simulink model "ss_feedback"  (R2022a)
settings: Solver=VariableStepAuto  StartTime=0.0  StopTime=100  RelTol=1e-3
values from neighbouring files (symbols this model uses):
  B = [0 2]'    [delayIndependent_Razumikhin_analysis.m]
  C = eye(2)    [delayIndependent_Razumikhin_synthesis.m]
  K = -[0.9 0]    [delayIndependent_Razumikhin_analysis.m]    (also in delayIndependent_Razumikhin_synthesis.m = Y*P)
undefined symbols (not defined in the file or in its folder): A
settings Model: Creator=aaron  LastModifiedBy=aaron

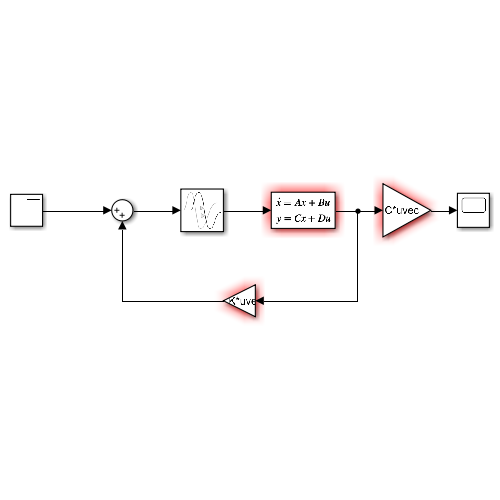
[thumbnail: Simulink's stored preview of the top-level diagram]
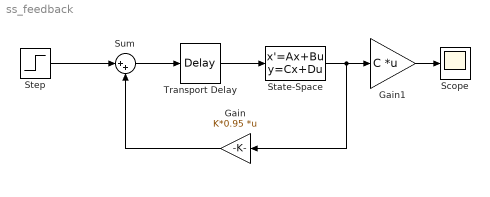
== system ss_feedback ==
  Gain : Gain  Gain=K*0.95  Multiplication=Matrix(K*u) (u vector)
  Gain1 : Gain  Gain=C  Multiplication=Matrix(K*u) (u vector)
  Scope : Scope
  State-Space : StateSpace  A=A  B=B  C=eye(2)  D=zeros(2,1)  InitialCondition=0
  Step : Step  Time=0  SampleTime=0
  Sum : Sum  Inputs=|++
  Transport Delay : TransportDelay  DelayTime=10
  wires:
  Transport Delay/1 -> State-Space/1
  State-Space/1 -> Gain/1, Gain1/1
  Step/1 -> Sum/1
  Sum/1 -> Transport Delay/1
  Gain/1 -> Sum/2
  Gain1/1 -> Scope/1
